simulink model "HDVPSG_DelayComp_NewRef_RealDrop_case1"  (R2019b)
settings: Solver=FixedStepDiscrete  StartTime=0.0  StopTime=28  FixedStep=UT.Ts_Veh  RelTol=1e-3
PostLoadFcn:
  | if any(exist('dsrtsu_mdlpostloadfcn', 'file') ~= 0), dsrtsu_mdlpostloadfcn('Execute', bdroot); end
InitFcn:
  | , if any(exist('dsmpb_private', 'file') ~= 0), dsmpb_private('dsmpb_mdlclblib', 'Init', bdroot); end,
values from neighbouring files (symbols this model uses):
  BETA_HDV_Leader = 50    [HDVPSG_DelayComp_NewRef_RealDrop_script_case1.m]
  BETA_PSG_Follower = 150    [HDVPSG_DelayComp_NewRef_RealDrop_script_case1.m]
  CtrlZone_Length = 250    [HDVPSG_DelayComp_NewRef_RealDrop_script_case1.m]
  DELTA_D_MIN = 5    [HDVPSG_DelayComp_NewRef_RealDrop_script_case1.m]
  DELTA_DR_MG_TCC = 15    [HDVPSG_DelayComp_NewRef_RealDrop_script_case1.m]
  HDV_AMAX = 1.3    [HDVPSG_DelayComp_NewRef_RealDrop_script_case1.m]
  HDV_AMIN = -2.5    [HDVPSG_DelayComp_NewRef_RealDrop_script_case1.m]
  HDV_first_v0 = 13    [HDVPSG_DelayComp_NewRef_RealDrop_script_case1.m]
  HDV_HighMu_D = 9    [HDVPSG_DelayComp_NewRef_RealDrop_script_case1.m]
  HDV_HighMu_I = 27    [HDVPSG_DelayComp_NewRef_RealDrop_script_case1.m]
  HDV_HighMu_P = 27    [HDVPSG_DelayComp_NewRef_RealDrop_script_case1.m]
  HDV_HighMu_TRFC = 0.7    [HDVPSG_DelayComp_NewRef_RealDrop_script_case1.m]
  HDV_last_v0 = 13    [HDVPSG_DelayComp_NewRef_RealDrop_script_case1.m]
  HDV_LowMu_D = 6    [HDVPSG_DelayComp_NewRef_RealDrop_script_case1.m]
  HDV_LowMu_I = 8    [HDVPSG_DelayComp_NewRef_RealDrop_script_case1.m]
  HDV_LowMu_P = 12    [HDVPSG_DelayComp_NewRef_RealDrop_script_case1.m]
  HDV_LowMu_TRFC = 0.6    [HDVPSG_DelayComp_NewRef_RealDrop_script_case1.m]
  Np_MPC = 20    [HDVPSG_DelayComp_NewRef_RealDrop_script_case1.m]
  PSG_AMAX = 3.2    [HDVPSG_DelayComp_NewRef_RealDrop_script_case1.m]
  PSG_AMIN = -6    [HDVPSG_DelayComp_NewRef_RealDrop_script_case1.m]
  PSG_end_v0 = 13    [HDVPSG_DelayComp_NewRef_RealDrop_script_case1.m]
  PSG_first_v0 = 13    [HDVPSG_DelayComp_NewRef_RealDrop_script_case1.m]
  PSG_HighMu_D = 15    [HDVPSG_DelayComp_NewRef_RealDrop_script_case1.m]
  PSG_HighMu_I = 125    [HDVPSG_DelayComp_NewRef_RealDrop_script_case1.m]
  PSG_HighMu_P = 75    [HDVPSG_DelayComp_NewRef_RealDrop_script_case1.m]
  PSG_HighMu_TRFC = 0.8    [HDVPSG_DelayComp_NewRef_RealDrop_script_case1.m]
  PSG_LowMu_D = 12    [HDVPSG_DelayComp_NewRef_RealDrop_script_case1.m]
  PSG_LowMu_I = 64    [HDVPSG_DelayComp_NewRef_RealDrop_script_case1.m]
  PSG_LowMu_P = 48    [HDVPSG_DelayComp_NewRef_RealDrop_script_case1.m]
  PSG_LowMu_TRFC = 0.7    [HDVPSG_DelayComp_NewRef_RealDrop_script_case1.m]
  PSG_middle_v0 = 13    [HDVPSG_DelayComp_NewRef_RealDrop_script_case1.m]
  Q_Leader = 1    [HDVPSG_DelayComp_NewRef_RealDrop_script_case1.m]
  Qd_dot_PSG_Follower = 2    [HDVPSG_DelayComp_NewRef_RealDrop_script_case1.m]
  Qd_PSG_Follower = 10    [HDVPSG_DelayComp_NewRef_RealDrop_script_case1.m]
  R_Leader = 20    [HDVPSG_DelayComp_NewRef_RealDrop_script_case1.m]
  R_PSG_Follower = 1    [HDVPSG_DelayComp_NewRef_RealDrop_script_case1.m]
  Recved_40_1 = Recved_Flag_Combined(47740,:)    [HDVPSG_DelayComp_NewRef_RealDrop_script_case1.m]
  Recved_40_2 = Recved_Flag_Combined(47780,:)    [HDVPSG_DelayComp_NewRef_RealDrop_script_case1.m]
  Recved_40_3 = Recved_Flag_Combined(49536,:)    [HDVPSG_DelayComp_NewRef_RealDrop_script_case1.m]
  Recved_40_4 = Recved_Flag_Combined(118106,:)    [HDVPSG_DelayComp_NewRef_RealDrop_script_case1.m]
  Rho_deltad_PSG_Follower = 1e3    (= 1000)    [HDVPSG_DelayComp_NewRef_RealDrop_script_case1.m]
  Rho_v_PSG_Follower = 1e3    (= 1000)    [HDVPSG_DelayComp_NewRef_RealDrop_script_case1.m]
  T_ADE = 0.01    [HDVPSG_DelayComp_NewRef_RealDrop_script_case1.m]
  V_MAX = 40    [HDVPSG_DelayComp_NewRef_RealDrop_script_case1.m]
  V_MIN = 0    [HDVPSG_DelayComp_NewRef_RealDrop_script_case1.m]
  VR_MG_TCC = 15    [HDVPSG_DelayComp_NewRef_RealDrop_script_case1.m]
undefined symbols (not defined in the file or in its folder): DiscIntNeverNeededParam, UT
libraries: simulink x46
(part 4 of 16)

== system HDVPSG_DelayComp_NewRef_RealDrop_case1/PSG2_control_withPDR_compen/Subsystem17 ==
  delta_dTCC : Inport
  T_end : Inport  Port=2
  veh0_dend_0 : Inport  Port=3
  veh2_dend_0 : Inport  Port=4
  veh0_v0 : Inport  Port=5
  veh2_v0 : Inport  Port=6
  Enable : EnablePort
  Add : Sum  Inputs=+-
  Add1 : Sum  Inputs=-+
  Poly_coefficient : MATLAB Function  TreatAsAtomicUnit=on
  a_0 : Outport
  a_1 : Outport  Port=2
  a_2 : Outport  Port=3
  a_3 : Outport  Port=4
  wires:
  Poly_coefficient/2(a_1) -> a_1/1
  Add/1 -> Poly_coefficient/1(delta_d0)
  Poly_coefficient/1(a_0) -> a_0/1
  T_end/1 -> Poly_coefficient/4(Tend)
  Add1/1 -> Poly_coefficient/3(delta_v0)  "delta_dr_dot"
  delta_dTCC/1 -> Poly_coefficient/2(delta_dTCC)
  Poly_coefficient/3(a_2) -> a_2/1
  Poly_coefficient/4(a_3) -> a_3/1
  veh0_dend_0/1 -> Add/2
  veh2_dend_0/1 -> Add/1
  veh2_v0/1 -> Add1/1
  veh0_v0/1 -> Add1/2

== system HDVPSG_DelayComp_NewRef_RealDrop_case1/PSG2_control_withPDR_compen/Subsystem18 ==
  a0 : Inport
  a1 : Inport  Port=2
  a2 : Inport  Port=3
  a3 : Inport  Port=4
  t_sumo : Inport  Port=5
  Ref : MATLAB Function  TreatAsAtomicUnit=on
  Ref_Pre_Vec : MATLAB Function  TreatAsAtomicUnit=on
  delta_dr : Outport
  delta_dr_dot : Outport  Port=2
  delta_dr_Pre_Vec : Outport  Port=3
  delta_dr_dot_Pre_Vec : Outport  Port=4
  wires:
  a2/1 -> Ref_Pre_Vec/3(a_2), Ref/3(a_2)
  Ref/2(delta_dr_dot) -> delta_dr_dot/1
  Ref/1(delta_dr) -> delta_dr/1
  t_sumo/1 -> Ref_Pre_Vec/5(t_sumo), Ref/5(t_sumo)
  a3/1 -> Ref_Pre_Vec/4(a_3), Ref/4(a_3)
  a1/1 -> Ref_Pre_Vec/2(a_1), Ref/2(a_1)
  a0/1 -> Ref_Pre_Vec/1(a_0), Ref/1(a_0)
  Ref_Pre_Vec/1(delta_dr_Pre_Vec) -> delta_dr_Pre_Vec/1
  Ref_Pre_Vec/2(delta_dr_dot_Pre_Vec) -> delta_dr_dot_Pre_Vec/1

== system HDVPSG_DelayComp_NewRef_RealDrop_case1/PSG2_control_withPDR_compen/Subsystem2 ==
  Lost_Step : Inport
  delta_d_pre_freeze_if_lost : Inport  Port=2
  delta_d_measure : Inport  Port=3
  Constant1 : Constant  Value=[1:1:Np_MPC+1]
  Lookup Table Dynamic : simulink/Lookup Tables/Lookup Table Dynamic  LookUpMeth=Interpolation-Extrapolation  OutDataType=fixdt('double')  OutScaling=[]  OutputDataTypeScalingMode=Specify via dialog  OutDataTypeStr=double  DoSatur=off
      settings: SourceProductName=Simulink
  MATLAB Function3 : MATLAB Function  TreatAsAtomicUnit=on
  Mux : Mux  Inputs=2
  Saturation : Saturate  UpperLimit=Np_MPC+1  LowerLimit=0
  Scope : Scope
  Switch : Switch  Criteria=u2 > Threshold  Threshold=Np_MPC+1
  delta_d_enhanced : Outport
  wires:
  delta_d_pre_freeze_if_lost/1 -> MATLAB Function3/2(delta_d_pre_freeze_if_lost), Lookup Table Dynamic/3
  delta_d_measure/1 -> MATLAB Function3/3(delta_d_measure)
  Constant1/1 -> Lookup Table Dynamic/2
  Lost_Step/1 -> Switch/2, Saturation/1, Lookup Table Dynamic/1
  Mux/1 -> Scope/1
  Switch/1 -> delta_d_enhanced/1
  Lookup Table Dynamic/1 -> Mux/1, Switch/1  "extrapolation_outside_Hp"
  MATLAB Function3/1(delta_d_MPC) -> Mux/2, Switch/3  "within Hp"
  Saturation/1 -> MATLAB Function3/1(Lost_Step)

== system HDVPSG_DelayComp_NewRef_RealDrop_case1/PSG2_control_withPDR_compen/Subsystem3 ==
  v_ego : Inport
  a_ego : Inport  Port=2
  t_all_leader : Inport  Port=3
  t_leader_has_run : Inport  Port=4
  Time_headway : Inport  Port=5
  t_PRE_has_run : Inport  Port=6
  Enable : EnablePort
  Add9 : Sum  Inputs=+-+
  v_ego_ini : Outport
  a_ego_ini : Outport  Port=2
  T_all_to_MP_ego : Outport  Port=3
  t_PRE_has_run_ini : Outport  Port=4
  wires:
  v_ego/1 -> v_ego_ini/1
  a_ego/1 -> a_ego_ini/1
  Add9/1 -> T_all_to_MP_ego/1
  t_leader_has_run/1 -> Add9/2
  Time_headway/1 -> Add9/3
  t_all_leader/1 -> Add9/1
  t_PRE_has_run/1 -> t_PRE_has_run_ini/1

== system HDVPSG_DelayComp_NewRef_RealDrop_case1/PSG3_control_withPDR_compen/Enabled and Triggered Subsystem ==
  delta_d_pre : Inport
  Enable : EnablePort
  delta_d_pre_freeze : Outport
  wires:
  delta_d_pre/1 -> delta_d_pre_freeze/1

== system HDVPSG_DelayComp_NewRef_RealDrop_case1/PSG3_control_withPDR_compen/Subsystem ==
  Recv : Inport
  Compare To Zero1 : simulink/Logic and Bit Operations/Compare To Zero  relop===  OutDataTypeStr=boolean
  Constant3 : Constant  Value=0
  Enabled and Triggered Subsystem1 : Subsystem  TreatAsAtomicUnit=on
  Switch : Switch  Criteria=u2 > Threshold
  Lost_Step : Outport
  wires:
  Switch/1 -> Lost_Step/1
  Recv/1 -> Compare To Zero1/1
  Constant3/1 -> Switch/3
  Enabled and Triggered Subsystem1/1(Lost_stop) -> Switch/1
  Compare To Zero1/1 -> Enabled and Triggered Subsystem1/Enable, Switch/2

== system HDVPSG_DelayComp_NewRef_RealDrop_case1/PSG3_control_withPDR_compen/Subsystem17 ==
  delta_dTCC : Inport
  T_end : Inport  Port=2
  veh0_dend_0 : Inport  Port=3
  veh2_dend_0 : Inport  Port=4
  veh0_v0 : Inport  Port=5
  veh2_v0 : Inport  Port=6
  Enable : EnablePort
  Add : Sum  Inputs=+-
  Add1 : Sum  Inputs=-+
  Poly_coefficient : MATLAB Function  TreatAsAtomicUnit=on
  a_0 : Outport
  a_1 : Outport  Port=2
  a_2 : Outport  Port=3
  a_3 : Outport  Port=4
  wires:
  veh0_v0/1 -> Add1/2
  veh2_v0/1 -> Add1/1
  veh2_dend_0/1 -> Add/1
  veh0_dend_0/1 -> Add/2
  Poly_coefficient/4(a_3) -> a_3/1
  Poly_coefficient/3(a_2) -> a_2/1
  delta_dTCC/1 -> Poly_coefficient/2(delta_dTCC)
  Add1/1 -> Poly_coefficient/3(delta_v0)  "delta_dr_dot"
  T_end/1 -> Poly_coefficient/4(Tend)
  Poly_coefficient/1(a_0) -> a_0/1
  Add/1 -> Poly_coefficient/1(delta_d0)
  Poly_coefficient/2(a_1) -> a_1/1

== system HDVPSG_DelayComp_NewRef_RealDrop_case1/PSG3_control_withPDR_compen/Subsystem18 ==
  a0 : Inport
  a1 : Inport  Port=2
  a2 : Inport  Port=3
  a3 : Inport  Port=4
  t_sumo : Inport  Port=5
  Ref : MATLAB Function  TreatAsAtomicUnit=on
  Ref_Pre_Vec : MATLAB Function  TreatAsAtomicUnit=on
  delta_dr : Outport
  delta_dr_dot : Outport  Port=2
  delta_dr_Pre_Vec : Outport  Port=3
  delta_dr_dot_Pre_Vec : Outport  Port=4
  wires:
  Ref_Pre_Vec/2(delta_dr_dot_Pre_Vec) -> delta_dr_dot_Pre_Vec/1
  Ref_Pre_Vec/1(delta_dr_Pre_Vec) -> delta_dr_Pre_Vec/1
  a0/1 -> Ref/1(a_0), Ref_Pre_Vec/1(a_0)
  a1/1 -> Ref/2(a_1), Ref_Pre_Vec/2(a_1)
  a3/1 -> Ref/4(a_3), Ref_Pre_Vec/4(a_3)
  t_sumo/1 -> Ref/5(t_sumo), Ref_Pre_Vec/5(t_sumo)
  Ref/1(delta_dr) -> delta_dr/1
  Ref/2(delta_dr_dot) -> delta_dr_dot/1
  a2/1 -> Ref/3(a_2), Ref_Pre_Vec/3(a_2)

== system HDVPSG_DelayComp_NewRef_RealDrop_case1/PSG3_control_withPDR_compen/Subsystem2 ==
  Lost_Step : Inport
  delta_d_pre_freeze_if_lost : Inport  Port=2
  delta_d_measure : Inport  Port=3
  Constant1 : Constant  Value=[1:1:Np_MPC+1]
  Lookup Table Dynamic : simulink/Lookup Tables/Lookup Table Dynamic  LookUpMeth=Interpolation-Extrapolation  OutDataType=fixdt('double')  OutScaling=[]  OutputDataTypeScalingMode=Specify via dialog  OutDataTypeStr=double  DoSatur=off
      settings: SourceProductName=Simulink
  MATLAB Function3 : MATLAB Function  TreatAsAtomicUnit=on
  Mux : Mux  Inputs=2
  Saturation : Saturate  UpperLimit=Np_MPC+1  LowerLimit=0
  Scope : Scope
  Switch : Switch  Criteria=u2 > Threshold  Threshold=Np_MPC+1
  delta_d_enhanced : Outport
  wires:
  delta_d_pre_freeze_if_lost/1 -> MATLAB Function3/2(delta_d_pre_freeze_if_lost), Lookup Table Dynamic/3
  delta_d_measure/1 -> MATLAB Function3/3(delta_d_measure)
  Constant1/1 -> Lookup Table Dynamic/2
  Lost_Step/1 -> Switch/2, Saturation/1, Lookup Table Dynamic/1
  Mux/1 -> Scope/1
  Switch/1 -> delta_d_enhanced/1
  Lookup Table Dynamic/1 -> Mux/1, Switch/1  "extrapolation_outside_Hp"
  MATLAB Function3/1(delta_d_MPC) -> Mux/2, Switch/3  "within Hp"
  Saturation/1 -> MATLAB Function3/1(Lost_Step)

== system HDVPSG_DelayComp_NewRef_RealDrop_case1/PSG3_control_withPDR_compen/Subsystem3 ==
  v_ego : Inport
  a_ego : Inport  Port=2
  t_all_leader : Inport  Port=3
  t_leader_has_run : Inport  Port=4
  Time_headway : Inport  Port=5
  t_PRE_has_run : Inport  Port=6
  Enable : EnablePort
  Add9 : Sum  Inputs=+-+
  v_ego_ini : Outport
  a_ego_ini : Outport  Port=2
  T_all_to_MP_ego : Outport  Port=3
  t_PRE_has_run_ini : Outport  Port=4
  wires:
  t_PRE_has_run/1 -> t_PRE_has_run_ini/1
  t_all_leader/1 -> Add9/1
  Time_headway/1 -> Add9/3
  t_leader_has_run/1 -> Add9/2
  Add9/1 -> T_all_to_MP_ego/1
  a_ego/1 -> a_ego_ini/1
  v_ego/1 -> v_ego_ini/1

== system HDVPSG_DelayComp_NewRef_RealDrop_case1/Subsystem1/PSG_first ==
  note: [v: 0--13--20]
      | High Frict PSG: P=75, I=125, D=15, TRFC=0.8 -->   -7.2<a<4.4
      | Low Frict  PSG: P=48, I=64,   D=12, TRFC=0.7 -->   -6.0<a<3.2
      |
      | High Frict HDV: P=27, I=27, D=9, TRFC=0.7 -->  -4.3<a<2.2
      | Low Frict  HDV: P=12, I=8,   D=6, TRFC=0.6 -->  -2.5<a<1.3
      |
      | ULMPC treat sudden drop of TRFC!
  vxr : Inport
  PID_P : Inport  Port=2
  PID_I : Inport  Port=3
  PID_D : Inport  Port=4
  TRFC : Inport  Port=5
  v_ini : Inport  Port=6
  Body Fixed Vehicle Dynamics : Subsystem
  Constant{1..5} (5 alike) : Constant  Value=0
  Cruise Speed Control : Subsystem
  Gain{,1..3} (4 alike) : Gain  Gain=UT.Rw
  Global Coordinates : Subsystem
  Scope : Scope
  Scope1 : Scope
  Scope3 : Scope
  Terminator : Terminator
  Vx : Scope
  X : Scope
  Y : Scope
  ax : Scope
  ay : Scope
  deg/rad : Gain  Gain=pi/180
  deg/rad1 : Gain  Gain=pi/180
  left/right wheel steer : Subsystem
  omegafl : Scope
  omegafr : Scope
  omegarl : Scope
  omegarr : Scope
  vy : Scope
  yaw : Scope
  yaw_rate : Scope
  vx : Outport
  wires:
  Constant4/1 -> Body Fixed Vehicle Dynamics/2(Brake)
  Constant3/1 -> Body Fixed Vehicle Dynamics/5(slope)
  Body Fixed Vehicle Dynamics/5(ax) -> ax/1
  Body Fixed Vehicle Dynamics/8(Yaw Angle) -> yaw/1, Global Coordinates/1(Heading Angle)
  left/right wheel steer/2(Left wheel steer ground (deg)) -> deg/rad/1
  left/right wheel steer/1(Right wheel steer ground (deg)) -> deg/rad1/1
  deg/rad1/1 -> Scope3/1, Body Fixed Vehicle Dynamics/3(deltaFR)
  Gain3/1 -> omegarr/1
  Global Coordinates/2(Y) -> Y/1
  Body Fixed Vehicle Dynamics/2(omegafr) -> Gain1/1
  Constant1/1 -> left/right wheel steer/1(steering wheel angle deg)
  deg/rad/1 -> Body Fixed Vehicle Dynamics/4(deltaFL)
  Body Fixed Vehicle Dynamics/11(Beta) -> Terminator/1
  Body Fixed Vehicle Dynamics/9(ay) -> ay/1
  Gain1/1 -> omegafr/1
  vxr/1 -> Cruise Speed Control/2(Vxr)
  Body Fixed Vehicle Dynamics/12(Sideslip Angle Alpha) -> Scope/1
  Body Fixed Vehicle Dynamics/7("Yaw Rate ") -> yaw_rate/1
  Gain/1 -> omegafl/1
  Gain2/1 -> omegarl/1
  Cruise Speed Control/1(Throttle) -> Body Fixed Vehicle Dynamics/1(Tdf), Scope1/1
  Body Fixed Vehicle Dynamics/10(Vy) -> Global Coordinates/3(Vy), vy/1
  Body Fixed Vehicle Dynamics/1(omegafl) -> Gain/1
  Body Fixed Vehicle Dynamics/4(omegarr) -> Gain3/1
  Body Fixed Vehicle Dynamics/3(omegarl) -> Gain2/1
  Body Fixed Vehicle Dynamics/6(Vx) -> Global Coordinates/2(Vx), Vx/1, Cruise Speed Control/1(Vx), vx/1
  Global Coordinates/1(X) -> X/1
  PID_P/1 -> Cruise Speed Control/3(PID_P)
  PID_I/1 -> Cruise Speed Control/4(PID_I)
  PID_D/1 -> Cruise Speed Control/5(PID_D)
  TRFC/1 -> Body Fixed Vehicle Dynamics/6(TRFC)
  v_ini/1 -> Body Fixed Vehicle Dynamics/7(V_ini)
  Constant2/1 -> Body Fixed Vehicle Dynamics/8(yaw_ini)
  Constant5/1 -> Body Fixed Vehicle Dynamics/9(vy_ini)

== system HDVPSG_DelayComp_NewRef_RealDrop_case1/Subsystem1/Subsystem4 ==
  Dist_to_MP : Inport
  Constant57 : Constant  Value=PSG_HighMu_P
  Constant58 : Constant  Value=PSG_LowMu_P
  MATLAB Function : MATLAB Function  TreatAsAtomicUnit=on
  Switch : Switch  Criteria=u2 > Threshold
  PSG_P : Outport
  HighMu : Outport  Port=2
  wires:
  MATLAB Function/1(HighTRFC) -> HighMu/1, Switch/2
  Dist_to_MP/1 -> MATLAB Function/1(distMP)
  Constant57/1 -> Switch/1
  Constant58/1 -> Switch/3
  Switch/1 -> PSG_P/1

== system HDVPSG_DelayComp_NewRef_RealDrop_case1/Subsystem1/Subsystem5 ==
  Dist_to_MP : Inport
  Constant57 : Constant  Value=PSG_HighMu_I
  Constant58 : Constant  Value=PSG_LowMu_I
  MATLAB Function : MATLAB Function  TreatAsAtomicUnit=on
  Switch : Switch  Criteria=u2 > Threshold
  PSG_I : Outport
  wires:
  Dist_to_MP/1 -> MATLAB Function/1(distMP)
  Switch/1 -> PSG_I/1
  Constant58/1 -> Switch/3
  Constant57/1 -> Switch/1
  MATLAB Function/1(HighTRFC) -> Switch/2

== system HDVPSG_DelayComp_NewRef_RealDrop_case1/Subsystem1/Subsystem6 ==
  Dist_to_MP : Inport
  Constant57 : Constant  Value=PSG_HighMu_D
  Constant58 : Constant  Value=PSG_LowMu_D
  MATLAB Function : MATLAB Function  TreatAsAtomicUnit=on
  Switch : Switch  Criteria=u2 > Threshold
  PSG_D : Outport
  wires:
  Dist_to_MP/1 -> MATLAB Function/1(distMP)
  Constant57/1 -> Switch/1
  Constant58/1 -> Switch/3
  Switch/1 -> PSG_D/1
  MATLAB Function/1(HighTRFC) -> Switch/2

== system HDVPSG_DelayComp_NewRef_RealDrop_case1/Subsystem1/Subsystem7 ==
  Dist_to_MP : Inport
  Constant1 : Constant  Value=PSG_LowMu_TRFC
  Constant57 : Constant  Value=PSG_HighMu_TRFC
  MATLAB Function : MATLAB Function  TreatAsAtomicUnit=on
  Switch : Switch  Criteria=u2 > Threshold
  PSG_Mu : Outport
  wires:
  Dist_to_MP/1 -> MATLAB Function/1(distMP)
  Switch/1 -> PSG_Mu/1
  Constant1/1 -> Switch/3
  Constant57/1 -> Switch/1
  MATLAB Function/1(HighTRFC) -> Switch/2

== system HDVPSG_DelayComp_NewRef_RealDrop_case1/Subsystem12/ARE_First_Order_Derivative_[1,0,0]5 ==
  a : Inport
  Trigger : TriggerPort  TriggerType=either  VariantControl=Variant  ZeroCross=off  PortDimensions=1
  Constant : Constant  Value=T_ADE
  Constant52 : Constant  Value=0
  MATLAB Function : MATLAB Function  TreatAsAtomicUnit=on
  a_dot_hat : Outport  VectorParamsAs1DForOutWhenUnconnected=off
  wires:
  Constant52/1 -> MATLAB Function/3(u_init)
  a/1 -> MATLAB Function/1(U)
  MATLAB Function/1(Dot_U) -> a_dot_hat/1
  Constant/1 -> MATLAB Function/2(Ts)

== system HDVPSG_DelayComp_NewRef_RealDrop_case1/Subsystem15/Enabled Subsystem1 ==
  Front_to_end : Inport
  Enable : EnablePort
  Front_to_end_PDR : Outport
  wires:
  Front_to_end/1 -> Front_to_end_PDR/1

== system HDVPSG_DelayComp_NewRef_RealDrop_case1/Subsystem15/Enabled Subsystem2 ==
  v_Front : Inport
  Enable : EnablePort
  v_Front_PDR : Outport
  wires:
  v_Front/1 -> v_Front_PDR/1

== system HDVPSG_DelayComp_NewRef_RealDrop_case1/Subsystem15/Enabled Subsystem3 ==
  a_Front : Inport
  Enable : EnablePort
  a_Front_PDR : Outport
  wires:
  a_Front/1 -> a_Front_PDR/1

== system HDVPSG_DelayComp_NewRef_RealDrop_case1/Subsystem2/PSG_first ==
  note: [v: 0--13--20]
      | High Frict PSG: P=75, I=125, D=15, TRFC=0.8 -->   -7.2<a<4.4
      | Low Frict  PSG: P=48, I=64,   D=12, TRFC=0.7 -->   -6.0<a<3.2
      |
      | High Frict HDV: P=27, I=27, D=9, TRFC=0.7 -->  -4.3<a<2.2
      | Low Frict  HDV: P=12, I=8,   D=6, TRFC=0.6 -->  -2.5<a<1.3
      |
      | ULMPC treat sudden drop of TRFC!
  vxr : Inport
  PID_P : Inport  Port=2
  PID_I : Inport  Port=3
  PID_D : Inport  Port=4
  TRFC : Inport  Port=5
  v_ini : Inport  Port=6
  Body Fixed Vehicle Dynamics : Subsystem
  Constant{1..5} (5 alike) : Constant  Value=0
  Cruise Speed Control : Subsystem
  Gain{,1..3} (4 alike) : Gain  Gain=UT.Rw
  Global Coordinates : Subsystem
  Scope : Scope
  Scope1 : Scope
  Scope3 : Scope
  Terminator : Terminator
  Vx : Scope
  X : Scope
  Y : Scope
  ax : Scope
  ay : Scope
  deg/rad : Gain  Gain=pi/180
  deg/rad1 : Gain  Gain=pi/180
  left/right wheel steer : Subsystem
  omegafl : Scope
  omegafr : Scope
  omegarl : Scope
  omegarr : Scope
  vy : Scope
  yaw : Scope
  yaw_rate : Scope
  vx : Outport
  wires:
  Constant5/1 -> Body Fixed Vehicle Dynamics/9(vy_ini)
  Constant2/1 -> Body Fixed Vehicle Dynamics/8(yaw_ini)
  v_ini/1 -> Body Fixed Vehicle Dynamics/7(V_ini)
  TRFC/1 -> Body Fixed Vehicle Dynamics/6(TRFC)
  PID_D/1 -> Cruise Speed Control/5(PID_D)
  PID_I/1 -> Cruise Speed Control/4(PID_I)
  PID_P/1 -> Cruise Speed Control/3(PID_P)
  Global Coordinates/1(X) -> X/1
  Body Fixed Vehicle Dynamics/6(Vx) -> vx/1, Cruise Speed Control/1(Vx), Vx/1, Global Coordinates/2(Vx)
  Body Fixed Vehicle Dynamics/3(omegarl) -> Gain2/1
  Body Fixed Vehicle Dynamics/4(omegarr) -> Gain3/1
  Body Fixed Vehicle Dynamics/1(omegafl) -> Gain/1
  Body Fixed Vehicle Dynamics/10(Vy) -> vy/1, Global Coordinates/3(Vy)
  Cruise Speed Control/1(Throttle) -> Scope1/1, Body Fixed Vehicle Dynamics/1(Tdf)
  Gain2/1 -> omegarl/1
  Gain/1 -> omegafl/1
  Body Fixed Vehicle Dynamics/7("Yaw Rate ") -> yaw_rate/1
  Body Fixed Vehicle Dynamics/12(Sideslip Angle Alpha) -> Scope/1
  vxr/1 -> Cruise Speed Control/2(Vxr)
  Gain1/1 -> omegafr/1
  Body Fixed Vehicle Dynamics/9(ay) -> ay/1
  Body Fixed Vehicle Dynamics/11(Beta) -> Terminator/1
  deg/rad/1 -> Body Fixed Vehicle Dynamics/4(deltaFL)
  Constant1/1 -> left/right wheel steer/1(steering wheel angle deg)
  Body Fixed Vehicle Dynamics/2(omegafr) -> Gain1/1
  Global Coordinates/2(Y) -> Y/1
  Gain3/1 -> omegarr/1
  deg/rad1/1 -> Body Fixed Vehicle Dynamics/3(deltaFR), Scope3/1
  left/right wheel steer/1(Right wheel steer ground (deg)) -> deg/rad1/1
  left/right wheel steer/2(Left wheel steer ground (deg)) -> deg/rad/1
  Body Fixed Vehicle Dynamics/8(Yaw Angle) -> Global Coordinates/1(Heading Angle), yaw/1
  Body Fixed Vehicle Dynamics/5(ax) -> ax/1
  Constant3/1 -> Body Fixed Vehicle Dynamics/5(slope)
  Constant4/1 -> Body Fixed Vehicle Dynamics/2(Brake)

== system HDVPSG_DelayComp_NewRef_RealDrop_case1/Subsystem2/Subsystem4 ==
  Dist_to_MP : Inport
  Constant57 : Constant  Value=PSG_HighMu_P
  Constant58 : Constant  Value=PSG_LowMu_P
  MATLAB Function : MATLAB Function  TreatAsAtomicUnit=on
  Switch : Switch  Criteria=u2 > Threshold
  PSG_P : Outport
  HighMu : Outport  Port=2
  wires:
  Switch/1 -> PSG_P/1
  Constant58/1 -> Switch/3
  Constant57/1 -> Switch/1
  Dist_to_MP/1 -> MATLAB Function/1(distMP)
  MATLAB Function/1(HighTRFC) -> HighMu/1, Switch/2

== system HDVPSG_DelayComp_NewRef_RealDrop_case1/Subsystem2/Subsystem5 ==
  Dist_to_MP : Inport
  Constant57 : Constant  Value=PSG_HighMu_I
  Constant58 : Constant  Value=PSG_LowMu_I
  MATLAB Function : MATLAB Function  TreatAsAtomicUnit=on
  Switch : Switch  Criteria=u2 > Threshold
  PSG_I : Outport
  wires:
  Constant57/1 -> Switch/1
  Constant58/1 -> Switch/3
  Switch/1 -> PSG_I/1
  Dist_to_MP/1 -> MATLAB Function/1(distMP)
  MATLAB Function/1(HighTRFC) -> Switch/2

== system HDVPSG_DelayComp_NewRef_RealDrop_case1/Subsystem2/Subsystem6 ==
  Dist_to_MP : Inport
  Constant57 : Constant  Value=PSG_HighMu_D
  Constant58 : Constant  Value=PSG_LowMu_D
  MATLAB Function : MATLAB Function  TreatAsAtomicUnit=on
  Switch : Switch  Criteria=u2 > Threshold
  PSG_D : Outport
  wires:
  Switch/1 -> PSG_D/1
  Constant58/1 -> Switch/3
  Constant57/1 -> Switch/1
  Dist_to_MP/1 -> MATLAB Function/1(distMP)
  MATLAB Function/1(HighTRFC) -> Switch/2

== system HDVPSG_DelayComp_NewRef_RealDrop_case1/Subsystem2/Subsystem7 ==
  Dist_to_MP : Inport
  Constant1 : Constant  Value=PSG_LowMu_TRFC
  Constant57 : Constant  Value=PSG_HighMu_TRFC
  MATLAB Function : MATLAB Function  TreatAsAtomicUnit=on
  Switch : Switch  Criteria=u2 > Threshold
  PSG_Mu : Outport
  wires:
  Constant57/1 -> Switch/1
  Constant1/1 -> Switch/3
  Switch/1 -> PSG_Mu/1
  Dist_to_MP/1 -> MATLAB Function/1(distMP)
  MATLAB Function/1(HighTRFC) -> Switch/2

== system HDVPSG_DelayComp_NewRef_RealDrop_case1/Subsystem29/PSG_first ==
  note: [v: 0--13--20]
      | High Frict PSG: P=75, I=125, D=15, TRFC=0.8 -->   -7.2<a<4.4
      | Low Frict  PSG: P=48, I=64,   D=12, TRFC=0.7 -->   -6.0<a<3.2
      |
      | High Frict HDV: P=27, I=27, D=9, TRFC=0.7 -->  -4.3<a<2.2
      | Low Frict  HDV: P=12, I=8,   D=6, TRFC=0.6 -->  -2.5<a<1.3
      |
      | ULMPC treat sudden drop of TRFC!
  vxr : Inport
  PID_P : Inport  Port=2
  PID_I : Inport  Port=3
  PID_D : Inport  Port=4
  TRFC : Inport  Port=5
  v_ini : Inport  Port=6
  Body Fixed Vehicle Dynamics : Subsystem
  Constant{1..5} (5 alike) : Constant  Value=0
  Cruise Speed Control : Subsystem
  Gain{,1..3} (4 alike) : Gain  Gain=UT.Rw
  Global Coordinates : Subsystem
  Scope : Scope
  Scope1 : Scope
  Scope3 : Scope
  Terminator : Terminator
  Vx : Scope
  X : Scope
  Y : Scope
  ax : Scope
  ay : Scope
  deg/rad : Gain  Gain=pi/180
  deg/rad1 : Gain  Gain=pi/180
  left/right wheel steer : Subsystem
  omegafl : Scope
  omegafr : Scope
  omegarl : Scope
  omegarr : Scope
  vy : Scope
  yaw : Scope
  yaw_rate : Scope
  vx : Outport
  wires:
  Constant5/1 -> Body Fixed Vehicle Dynamics/9(vy_ini)
  Constant2/1 -> Body Fixed Vehicle Dynamics/8(yaw_ini)
  v_ini/1 -> Body Fixed Vehicle Dynamics/7(V_ini)
  TRFC/1 -> Body Fixed Vehicle Dynamics/6(TRFC)
  PID_D/1 -> Cruise Speed Control/5(PID_D)
  PID_I/1 -> Cruise Speed Control/4(PID_I)
  PID_P/1 -> Cruise Speed Control/3(PID_P)
  Global Coordinates/1(X) -> X/1
  Body Fixed Vehicle Dynamics/6(Vx) -> vx/1, Cruise Speed Control/1(Vx), Vx/1, Global Coordinates/2(Vx)
  Body Fixed Vehicle Dynamics/3(omegarl) -> Gain2/1
  Body Fixed Vehicle Dynamics/4(omegarr) -> Gain3/1
  Body Fixed Vehicle Dynamics/1(omegafl) -> Gain/1
  Body Fixed Vehicle Dynamics/10(Vy) -> vy/1, Global Coordinates/3(Vy)
  Cruise Speed Control/1(Throttle) -> Scope1/1, Body Fixed Vehicle Dynamics/1(Tdf)
  Gain2/1 -> omegarl/1
  Gain/1 -> omegafl/1
  Body Fixed Vehicle Dynamics/7("Yaw Rate ") -> yaw_rate/1
  Body Fixed Vehicle Dynamics/12(Sideslip Angle Alpha) -> Scope/1
  vxr/1 -> Cruise Speed Control/2(Vxr)
  Gain1/1 -> omegafr/1
  Body Fixed Vehicle Dynamics/9(ay) -> ay/1
  Body Fixed Vehicle Dynamics/11(Beta) -> Terminator/1
  deg/rad/1 -> Body Fixed Vehicle Dynamics/4(deltaFL)
  Constant1/1 -> left/right wheel steer/1(steering wheel angle deg)
  Body Fixed Vehicle Dynamics/2(omegafr) -> Gain1/1
  Global Coordinates/2(Y) -> Y/1
  Gain3/1 -> omegarr/1
  deg/rad1/1 -> Body Fixed Vehicle Dynamics/3(deltaFR), Scope3/1
  left/right wheel steer/1(Right wheel steer ground (deg)) -> deg/rad1/1
  left/right wheel steer/2(Left wheel steer ground (deg)) -> deg/rad/1
  Body Fixed Vehicle Dynamics/8(Yaw Angle) -> Global Coordinates/1(Heading Angle), yaw/1
  Body Fixed Vehicle Dynamics/5(ax) -> ax/1
  Constant3/1 -> Body Fixed Vehicle Dynamics/5(slope)
  Constant4/1 -> Body Fixed Vehicle Dynamics/2(Brake)

== system HDVPSG_DelayComp_NewRef_RealDrop_case1/Subsystem29/Subsystem4 ==
  Dist_to_MP : Inport
  Constant57 : Constant  Value=PSG_HighMu_P
  Constant58 : Constant  Value=PSG_LowMu_P
  MATLAB Function : MATLAB Function  TreatAsAtomicUnit=on
  Switch : Switch  Criteria=u2 > Threshold
  PSG_P : Outport
  HighMu : Outport  Port=2
  wires:
  Switch/1 -> PSG_P/1
  Constant58/1 -> Switch/3
  Constant57/1 -> Switch/1
  Dist_to_MP/1 -> MATLAB Function/1(distMP)
  MATLAB Function/1(HighTRFC) -> HighMu/1, Switch/2

== system HDVPSG_DelayComp_NewRef_RealDrop_case1/Subsystem29/Subsystem5 ==
  Dist_to_MP : Inport
  Constant57 : Constant  Value=PSG_HighMu_I
  Constant58 : Constant  Value=PSG_LowMu_I
  MATLAB Function : MATLAB Function  TreatAsAtomicUnit=on
  Switch : Switch  Criteria=u2 > Threshold
  PSG_I : Outport
  wires:
  Constant57/1 -> Switch/1
  Constant58/1 -> Switch/3
  Switch/1 -> PSG_I/1
  Dist_to_MP/1 -> MATLAB Function/1(distMP)
  MATLAB Function/1(HighTRFC) -> Switch/2

== system HDVPSG_DelayComp_NewRef_RealDrop_case1/Subsystem29/Subsystem6 ==
  Dist_to_MP : Inport
  Constant57 : Constant  Value=PSG_HighMu_D
  Constant58 : Constant  Value=PSG_LowMu_D
  MATLAB Function : MATLAB Function  TreatAsAtomicUnit=on
  Switch : Switch  Criteria=u2 > Threshold
  PSG_D : Outport
  wires:
  Switch/1 -> PSG_D/1
  Constant58/1 -> Switch/3
  Constant57/1 -> Switch/1
  Dist_to_MP/1 -> MATLAB Function/1(distMP)
  MATLAB Function/1(HighTRFC) -> Switch/2

== system HDVPSG_DelayComp_NewRef_RealDrop_case1/Subsystem29/Subsystem7 ==
  Dist_to_MP : Inport
  Constant1 : Constant  Value=PSG_LowMu_TRFC
  Constant57 : Constant  Value=PSG_HighMu_TRFC
  MATLAB Function : MATLAB Function  TreatAsAtomicUnit=on
  Switch : Switch  Criteria=u2 > Threshold
  PSG_Mu : Outport
  wires:
  Constant57/1 -> Switch/1
  Constant1/1 -> Switch/3
  Switch/1 -> PSG_Mu/1
  Dist_to_MP/1 -> MATLAB Function/1(distMP)
  MATLAB Function/1(HighTRFC) -> Switch/2

== system HDVPSG_DelayComp_NewRef_RealDrop_case1/Subsystem3/HDV_first ==
  note: [v: 0--13--20]
      | High Frict PSG: P=75, I=125, D=15, TRFC=0.8 -->   -7.2<a<4.4
      | Low Frict  PSG: P=48, I=64,   D=12, TRFC=0.7 -->   -6.0<a<3.2
      |
      | High Frict HDV: P=27, I=27, D=9, TRFC=0.7 -->  -4.3<a<2.2
      | Low Frict  HDV: P=12, I=8,   D=6, TRFC=0.6 -->  -2.5<a<1.3
      |
      | ULMPC treat sudden drop of TRFC!
  vxr : Inport
  PID_P : Inport  Port=2
  PID_I : Inport  Port=3
  PID_D : Inport  Port=4
  TRFC : Inport  Port=5
  v_ini : Inport  Port=6
  Body Fixed Vehicle Dynamics : Subsystem
  Constant{1..5} (5 alike) : Constant  Value=0
  Cruise Speed Control : Subsystem
  Gain{,1..3} (4 alike) : Gain  Gain=UT.Rw
  Global Coordinates : Subsystem
  Scope : Scope
  Scope1 : Scope
  Scope3 : Scope
  Terminator : Terminator
  Vx : Scope
  X : Scope
  Y : Scope
  ax : Scope
  ay : Scope
  deg/rad : Gain  Gain=pi/180
  deg/rad1 : Gain  Gain=pi/180
  left/right wheel steer : Subsystem
  omegafl : Scope
  omegafr : Scope
  omegarl : Scope
  omegarr : Scope
  vy : Scope
  yaw : Scope
  yaw_rate : Scope
  vx : Outport
  wires:
  Constant5/1 -> Body Fixed Vehicle Dynamics/9(vy_ini)
  Constant2/1 -> Body Fixed Vehicle Dynamics/8(yaw_ini)
  v_ini/1 -> Body Fixed Vehicle Dynamics/7(V_ini)
  TRFC/1 -> Body Fixed Vehicle Dynamics/6(TRFC)
  PID_D/1 -> Cruise Speed Control/5(PID_D)
  PID_I/1 -> Cruise Speed Control/4(PID_I)
  PID_P/1 -> Cruise Speed Control/3(PID_P)
  Global Coordinates/1(X) -> X/1
  Body Fixed Vehicle Dynamics/6(Vx) -> vx/1, Cruise Speed Control/1(Vx), Vx/1, Global Coordinates/2(Vx)
  Body Fixed Vehicle Dynamics/3(omegarl) -> Gain2/1
  Body Fixed Vehicle Dynamics/4(omegarr) -> Gain3/1
  Body Fixed Vehicle Dynamics/1(omegafl) -> Gain/1
  Body Fixed Vehicle Dynamics/10(Vy) -> vy/1, Global Coordinates/3(Vy)
  Cruise Speed Control/1(Throttle) -> Scope1/1, Body Fixed Vehicle Dynamics/1(Tdf)
  Gain2/1 -> omegarl/1
  Gain/1 -> omegafl/1
  Body Fixed Vehicle Dynamics/7("Yaw Rate ") -> yaw_rate/1
  Body Fixed Vehicle Dynamics/12(Sideslip Angle Alpha) -> Scope/1
  vxr/1 -> Cruise Speed Control/2(Vxr)
  Gain1/1 -> omegafr/1
  Body Fixed Vehicle Dynamics/9(ay) -> ay/1
  Body Fixed Vehicle Dynamics/11(Beta) -> Terminator/1
  deg/rad/1 -> Body Fixed Vehicle Dynamics/4(deltaFL)
  Constant1/1 -> left/right wheel steer/1(steering wheel angle deg)
  Body Fixed Vehicle Dynamics/2(omegafr) -> Gain1/1
  Global Coordinates/2(Y) -> Y/1
  Gain3/1 -> omegarr/1
  deg/rad1/1 -> Body Fixed Vehicle Dynamics/3(deltaFR), Scope3/1
  left/right wheel steer/1(Right wheel steer ground (deg)) -> deg/rad1/1
  left/right wheel steer/2(Left wheel steer ground (deg)) -> deg/rad/1
  Body Fixed Vehicle Dynamics/8(Yaw Angle) -> Global Coordinates/1(Heading Angle), yaw/1
  Body Fixed Vehicle Dynamics/5(ax) -> ax/1
  Constant3/1 -> Body Fixed Vehicle Dynamics/5(slope)
  Constant4/1 -> Body Fixed Vehicle Dynamics/2(Brake)

== system HDVPSG_DelayComp_NewRef_RealDrop_case1/Subsystem3/Subsystem16 ==
  Dist_to_MP : Inport
  Constant57 : Constant  Value=HDV_HighMu_P
  Constant58 : Constant  Value=HDV_LowMu_P
  MATLAB Function : MATLAB Function  TreatAsAtomicUnit=on
  Switch : Switch  Criteria=u2 > Threshold
  HDV_P : Outport
  HighMu : Outport  Port=2
  wires:
  Dist_to_MP/1 -> MATLAB Function/1(distMP)
  Constant58/1 -> Switch/3
  MATLAB Function/1(HighTRFC) -> HighMu/1, Switch/2
  Constant57/1 -> Switch/1
  Switch/1 -> HDV_P/1

== system HDVPSG_DelayComp_NewRef_RealDrop_case1/Subsystem3/Subsystem17 ==
  Dist_to_MP : Inport
  Constant57 : Constant  Value=HDV_HighMu_I
  Constant58 : Constant  Value=HDV_LowMu_I
  MATLAB Function : MATLAB Function  TreatAsAtomicUnit=on
  Switch : Switch  Criteria=u2 > Threshold
  HDV_I : Outport
  wires:
  MATLAB Function/1(HighTRFC) -> Switch/2
  Dist_to_MP/1 -> MATLAB Function/1(distMP)
  Constant58/1 -> Switch/3
  Constant57/1 -> Switch/1
  Switch/1 -> HDV_I/1

== system HDVPSG_DelayComp_NewRef_RealDrop_case1/Subsystem3/Subsystem18 ==
  Dist_to_MP : Inport
  Constant57 : Constant  Value=HDV_HighMu_D
  Constant58 : Constant  Value=HDV_LowMu_D
  MATLAB Function : MATLAB Function  TreatAsAtomicUnit=on
  Switch : Switch  Criteria=u2 > Threshold
  HDV_D : Outport
  wires:
  MATLAB Function/1(HighTRFC) -> Switch/2
  Dist_to_MP/1 -> MATLAB Function/1(distMP)
  Constant58/1 -> Switch/3
  Constant57/1 -> Switch/1
  Switch/1 -> HDV_D/1

== system HDVPSG_DelayComp_NewRef_RealDrop_case1/Subsystem3/Subsystem7 ==
  Dist_to_MP : Inport
  Constant1 : Constant  Value=HDV_LowMu_TRFC
  Constant57 : Constant  Value=HDV_HighMu_TRFC
  MATLAB Function : MATLAB Function  TreatAsAtomicUnit=on
  Switch : Switch  Criteria=u2 > Threshold
  HDV_Mu : Outport
  wires:
  MATLAB Function/1(HighTRFC) -> Switch/2
  Dist_to_MP/1 -> MATLAB Function/1(distMP)
  Constant1/1 -> Switch/3
  Constant57/1 -> Switch/1
  Switch/1 -> HDV_Mu/1

== system HDVPSG_DelayComp_NewRef_RealDrop_case1/Subsystem4/Enabled Subsystem1 ==
  Front_to_end : Inport
  Enable : EnablePort
  Front_to_end_PDR : Outport
  wires:
  Front_to_end/1 -> Front_to_end_PDR/1

== system HDVPSG_DelayComp_NewRef_RealDrop_case1/Subsystem4/Enabled Subsystem2 ==
  v_Front : Inport
  Enable : EnablePort
  v_Front_PDR : Outport
  wires:
  v_Front/1 -> v_Front_PDR/1

== system HDVPSG_DelayComp_NewRef_RealDrop_case1/Subsystem4/Enabled Subsystem3 ==
  a_Front : Inport
  Enable : EnablePort
  a_Front_PDR : Outport
  wires:
  a_Front/1 -> a_Front_PDR/1

== system HDVPSG_DelayComp_NewRef_RealDrop_case1/Subsystem5/Enabled Subsystem1 ==
  Front_to_end : Inport
  Enable : EnablePort
  Front_to_end_PDR : Outport
  wires:
  Front_to_end/1 -> Front_to_end_PDR/1

== system HDVPSG_DelayComp_NewRef_RealDrop_case1/Subsystem5/Enabled Subsystem2 ==
  v_Front : Inport
  Enable : EnablePort
  v_Front_PDR : Outport
  wires:
  v_Front/1 -> v_Front_PDR/1

== system HDVPSG_DelayComp_NewRef_RealDrop_case1/Subsystem5/Enabled Subsystem3 ==
  a_Front : Inport
  Enable : EnablePort
  a_Front_PDR : Outport
  wires:
  a_Front/1 -> a_Front_PDR/1

== system HDVPSG_DelayComp_NewRef_RealDrop_case1/Subsystem6/HDV_first ==
  note: [v: 0--13--20]
      | High Frict PSG: P=75, I=125, D=15, TRFC=0.8 -->   -7.2<a<4.4
      | Low Frict  PSG: P=48, I=64,   D=12, TRFC=0.7 -->   -6.0<a<3.2
      |
      | High Frict HDV: P=27, I=27, D=9, TRFC=0.7 -->  -4.3<a<2.2
      | Low Frict  HDV: P=12, I=8,   D=6, TRFC=0.6 -->  -2.5<a<1.3
      |
      | ULMPC treat sudden drop of TRFC!
  vxr : Inport
  PID_P : Inport  Port=2
  PID_I : Inport  Port=3
  PID_D : Inport  Port=4
  TRFC : Inport  Port=5
  v_ini : Inport  Port=6
  Body Fixed Vehicle Dynamics : Subsystem
  Constant{1..5} (5 alike) : Constant  Value=0
  Cruise Speed Control : Subsystem
  Gain{,1..3} (4 alike) : Gain  Gain=UT.Rw
  Global Coordinates : Subsystem
  Scope : Scope
  Scope1 : Scope
  Scope3 : Scope
  Terminator : Terminator
  Vx : Scope
  X : Scope
  Y : Scope
  ax : Scope
  ay : Scope
  deg/rad : Gain  Gain=pi/180
  deg/rad1 : Gain  Gain=pi/180
  left/right wheel steer : Subsystem
  omegafl : Scope
  omegafr : Scope
  omegarl : Scope
  omegarr : Scope
  vy : Scope
  yaw : Scope
  yaw_rate : Scope
  vx : Outport
  wires:
  Constant4/1 -> Body Fixed Vehicle Dynamics/2(Brake)
  Constant3/1 -> Body Fixed Vehicle Dynamics/5(slope)
  Body Fixed Vehicle Dynamics/5(ax) -> ax/1
  Body Fixed Vehicle Dynamics/8(Yaw Angle) -> yaw/1, Global Coordinates/1(Heading Angle)
  left/right wheel steer/2(Left wheel steer ground (deg)) -> deg/rad/1
  left/right wheel steer/1(Right wheel steer ground (deg)) -> deg/rad1/1
  deg/rad1/1 -> Scope3/1, Body Fixed Vehicle Dynamics/3(deltaFR)
  Gain3/1 -> omegarr/1
  Global Coordinates/2(Y) -> Y/1
  Body Fixed Vehicle Dynamics/2(omegafr) -> Gain1/1
  Constant1/1 -> left/right wheel steer/1(steering wheel angle deg)
  deg/rad/1 -> Body Fixed Vehicle Dynamics/4(deltaFL)
  Body Fixed Vehicle Dynamics/11(Beta) -> Terminator/1
  Body Fixed Vehicle Dynamics/9(ay) -> ay/1
  Gain1/1 -> omegafr/1
  vxr/1 -> Cruise Speed Control/2(Vxr)
  Body Fixed Vehicle Dynamics/12(Sideslip Angle Alpha) -> Scope/1
  Body Fixed Vehicle Dynamics/7("Yaw Rate ") -> yaw_rate/1
  Gain/1 -> omegafl/1
  Gain2/1 -> omegarl/1
  Cruise Speed Control/1(Throttle) -> Body Fixed Vehicle Dynamics/1(Tdf), Scope1/1
  Body Fixed Vehicle Dynamics/10(Vy) -> Global Coordinates/3(Vy), vy/1
  Body Fixed Vehicle Dynamics/1(omegafl) -> Gain/1
  Body Fixed Vehicle Dynamics/4(omegarr) -> Gain3/1
  Body Fixed Vehicle Dynamics/3(omegarl) -> Gain2/1
  Body Fixed Vehicle Dynamics/6(Vx) -> Global Coordinates/2(Vx), Vx/1, Cruise Speed Control/1(Vx), vx/1
  Global Coordinates/1(X) -> X/1
  PID_P/1 -> Cruise Speed Control/3(PID_P)
  PID_I/1 -> Cruise Speed Control/4(PID_I)
  PID_D/1 -> Cruise Speed Control/5(PID_D)
  TRFC/1 -> Body Fixed Vehicle Dynamics/6(TRFC)
  v_ini/1 -> Body Fixed Vehicle Dynamics/7(V_ini)
  Constant2/1 -> Body Fixed Vehicle Dynamics/8(yaw_ini)
  Constant5/1 -> Body Fixed Vehicle Dynamics/9(vy_ini)

== system HDVPSG_DelayComp_NewRef_RealDrop_case1/Subsystem6/Subsystem16 ==
  Dist_to_MP : Inport
  Constant57 : Constant  Value=HDV_HighMu_P
  Constant58 : Constant  Value=HDV_LowMu_P
  MATLAB Function : MATLAB Function  TreatAsAtomicUnit=on
  Switch : Switch  Criteria=u2 > Threshold
  HDV_P : Outport
  HighMu : Outport  Port=2
  wires:
  Constant58/1 -> Switch/3
  Dist_to_MP/1 -> MATLAB Function/1(distMP)
  MATLAB Function/1(HighTRFC) -> Switch/2, HighMu/1
  Constant57/1 -> Switch/1
  Switch/1 -> HDV_P/1

== system HDVPSG_DelayComp_NewRef_RealDrop_case1/Subsystem6/Subsystem17 ==
  Dist_to_MP : Inport
  Constant57 : Constant  Value=HDV_HighMu_I
  Constant58 : Constant  Value=HDV_LowMu_I
  MATLAB Function : MATLAB Function  TreatAsAtomicUnit=on
  Switch : Switch  Criteria=u2 > Threshold
  HDV_I : Outport
  wires:
  Constant58/1 -> Switch/3
  Dist_to_MP/1 -> MATLAB Function/1(distMP)
  MATLAB Function/1(HighTRFC) -> Switch/2
  Constant57/1 -> Switch/1
  Switch/1 -> HDV_I/1

== system HDVPSG_DelayComp_NewRef_RealDrop_case1/Subsystem6/Subsystem18 ==
  Dist_to_MP : Inport
  Constant57 : Constant  Value=HDV_HighMu_D
  Constant58 : Constant  Value=HDV_LowMu_D
  MATLAB Function : MATLAB Function  TreatAsAtomicUnit=on
  Switch : Switch  Criteria=u2 > Threshold
  HDV_D : Outport
  wires:
  Constant58/1 -> Switch/3
  Dist_to_MP/1 -> MATLAB Function/1(distMP)
  MATLAB Function/1(HighTRFC) -> Switch/2
  Constant57/1 -> Switch/1
  Switch/1 -> HDV_D/1

== system HDVPSG_DelayComp_NewRef_RealDrop_case1/Subsystem6/Subsystem7 ==
  Dist_to_MP : Inport
  Constant1 : Constant  Value=HDV_LowMu_TRFC
  Constant57 : Constant  Value=HDV_HighMu_TRFC
  MATLAB Function : MATLAB Function  TreatAsAtomicUnit=on
  Switch : Switch  Criteria=u2 > Threshold
  HDV_Mu : Outport
  wires:
  Constant1/1 -> Switch/3
  Dist_to_MP/1 -> MATLAB Function/1(distMP)
  MATLAB Function/1(HighTRFC) -> Switch/2
  Constant57/1 -> Switch/1
  Switch/1 -> HDV_Mu/1

== system HDVPSG_DelayComp_NewRef_RealDrop_case1/Subsystem7/Enabled Subsystem1 ==
  Front_to_end : Inport
  Enable : EnablePort
  Front_to_end_PDR : Outport
  wires:
  Front_to_end/1 -> Front_to_end_PDR/1

== system HDVPSG_DelayComp_NewRef_RealDrop_case1/Subsystem7/Enabled Subsystem2 ==
  v_Front : Inport
  Enable : EnablePort
  v_Front_PDR : Outport
  wires:
  v_Front/1 -> v_Front_PDR/1

== system HDVPSG_DelayComp_NewRef_RealDrop_case1/Subsystem7/Enabled Subsystem3 ==
  a_Front : Inport
  Enable : EnablePort
  a_Front_PDR : Outport
  wires:
  a_Front/1 -> a_Front_PDR/1

== system HDVPSG_DelayComp_NewRef_RealDrop_case1/HDV2_control_withPDR_compen/Subsystem/Enabled and Triggered Subsystem1 ==
  Enable : EnablePort  StatesWhenEnabling=reset
  Add : Sum
  Constant : Constant  SampleTime=T_ADE
  Memory : Memory
  Lost_stop : Outport
  wires:
  Constant/1 -> Add/1
  Memory/1 -> Add/2
  Add/1 -> Lost_stop/1, Memory/1

== system HDVPSG_DelayComp_NewRef_RealDrop_case1/PSG1_control_withPDR_compen/Subsystem/Enabled and Triggered Subsystem1 ==
  Enable : EnablePort  StatesWhenEnabling=reset
  Add : Sum
  Constant : Constant  SampleTime=T_ADE
  Memory : Memory
  Lost_stop : Outport
  wires:
  Add/1 -> Memory/1, Lost_stop/1
  Memory/1 -> Add/2
  Constant/1 -> Add/1

== system HDVPSG_DelayComp_NewRef_RealDrop_case1/PSG2_control_withPDR_compen/Subsystem/Enabled and Triggered Subsystem1 ==
  Enable : EnablePort  StatesWhenEnabling=reset
  Add : Sum
  Constant : Constant  SampleTime=T_ADE
  Memory : Memory
  Lost_stop : Outport
  wires:
  Constant/1 -> Add/1
  Memory/1 -> Add/2
  Add/1 -> Lost_stop/1, Memory/1

== system HDVPSG_DelayComp_NewRef_RealDrop_case1/PSG3_control_withPDR_compen/Subsystem/Enabled and Triggered Subsystem1 ==
  Enable : EnablePort  StatesWhenEnabling=reset
  Add : Sum
  Constant : Constant  SampleTime=T_ADE
  Memory : Memory
  Lost_stop : Outport
  wires:
  Add/1 -> Memory/1, Lost_stop/1
  Memory/1 -> Add/2
  Constant/1 -> Add/1

== system HDVPSG_DelayComp_NewRef_RealDrop_case1/Subsystem1/PSG_first/Body Fixed Vehicle Dynamics ==
  Tdf : Inport
  Brake : Inport  Port=2
  deltaFR : Inport  Port=3
  deltaFL : Inport  Port=4
  slope : Inport  Port=5
  TRFC : Inport  Port=6
  V_ini : Inport  Port=7
  yaw_ini : Inport  Port=8
  vy_ini : Inport  Port=9
  8dof_vehicle : Subsystem
  Brakes : Subsystem
  Bus Creator{,2..4} (4 alike) : BusCreator  Inputs=4
  Bus Creator1 : BusCreator  Inputs=8
  Bus Creator5 : BusCreator  Inputs=3
  Bus Selector : BusSelector  OutputSignals=signal1,signal2,signal3,signal4
  Constant : Constant  Value=0
  Constant1 : Constant  Value=0
  Driving Resistance Subsystem : Subsystem
  Fz : Subsystem
  Magic Formula Tire Model1 : Subsystem
  "Tire Longitudinal Center Speed " : Subsystem
  Tire Sideslip Angle : Subsystem
  Unit Delay : UnitDelay  SampleTime=UT.Ts_Veh  HasFrameUpgradeWarning=on
  Unit Delay1 : UnitDelay  SampleTime=UT.Ts_Veh  HasFrameUpgradeWarning=on
  deltaFL1 : InportShadow  Port=4
  deltaFL2 : InportShadow  Port=4
  deltaFR1 : InportShadow  Port=3
  deltaFR2 : InportShadow  Port=3
  lamda slip ratio : Subsystem
  omegafl : Outport  VectorParamsAs1DForOutWhenUnconnected=off
  omegafr : Outport  Port=2  VectorParamsAs1DForOutWhenUnconnected=off
  omegarl : Outport  Port=3  VectorParamsAs1DForOutWhenUnconnected=off
  omegarr : Outport  Port=4  VectorParamsAs1DForOutWhenUnconnected=off
  ax : Outport  Port=5  VectorParamsAs1DForOutWhenUnconnected=off
  Vx : Outport  Port=6  VectorParamsAs1DForOutWhenUnconnected=off
  "Yaw Rate " : Outport  Port=7  VectorParamsAs1DForOutWhenUnconnected=off
  Yaw Angle : Outport  Port=8  VectorParamsAs1DForOutWhenUnconnected=off
  ay : Outport  Port=9  VectorParamsAs1DForOutWhenUnconnected=off
  Vy : Outport  Port=10  VectorParamsAs1DForOutWhenUnconnected=off
  Beta : Outport  Port=11  VectorParamsAs1DForOutWhenUnconnected=off
  Sideslip Angle Alpha : Outport  Port=12  VectorParamsAs1DForOutWhenUnconnected=off
  wires:
  Brakes/4(Tbrr) -> 8dof_vehicle/5(Tbrr)
  Brakes/3(Tbrl) -> 8dof_vehicle/4(Tbrl)
  Brakes/2(Tbfr) -> 8dof_vehicle/3(Tbfr)
  Brakes/1(Tbfl) -> 8dof_vehicle/2(Tbfl)
  Brake/1 -> Brakes/2(brake postion)
  8dof_vehicle/14("Roll ") -> Fz/7(roll angle)
  8dof_vehicle/12(Pitch) -> Fz/4(pitch angle)
  8dof_vehicle/13(Pitch_rate) -> Fz/8(pitch rate)
  Bus Creator3/1 -> Bus Creator5/2
  deltaFR2/1 -> 8dof_vehicle/11(deltaRL)
  deltaFR1/1 -> Tire Sideslip Angle/5(deltaFR1)
  deltaFR/1 -> lamda slip ratio/10(deltaFR)
  lamda slip ratio/4(lamdarr) -> Bus Creator2/4
  lamda slip ratio/3(lamdarl) -> Bus Creator2/3
  lamda slip ratio/2(lamdafr) -> Bus Creator2/2
  lamda slip ratio/1(lamdafl) -> Bus Creator2/1
  Unit Delay/1 -> Fz/2(ax)
  Unit Delay1/1 -> Fz/5(ay)
  Magic Formula Tire Model1/4(Fy_FR) -> Bus Creator1/4
  Magic Formula Tire Model1/3(Fx_FR) -> Bus Creator1/3
  Magic Formula Tire Model1/6(Fy_RL) -> Bus Creator1/6
  Magic Formula Tire Model1/8(Fy_RR) -> Bus Creator1/8
  Magic Formula Tire Model1/7(Fx_RR) -> Bus Creator1/7
  Magic Formula Tire Model1/5(Fx_RL) -> Bus Creator1/5
  deltaFL2/1 -> 8dof_vehicle/10(deltaFL)  "deltaw"
  8dof_vehicle/5(ax) -> Unit Delay/1, ax/1
  Constant/1 -> Fz/3(slope)
  Driving Resistance Subsystem/1(Fax) -> 8dof_vehicle/7(Fax), Fz/1(Fa)
  Constant1/1 -> Fz/6(bank angle)
  slope/1 -> 8dof_vehicle/9(slope)
  8dof_vehicle/7(Yaw Rate) -> "Tire Longitudinal Center Speed "/3(YawRate), Tire Sideslip Angle/2(Yaw Rate), "Yaw Rate "/1
  8dof_vehicle/6(Vx) -> "Tire Longitudinal Center Speed "/1(Vx), Tire Sideslip Angle/3(Vx), Driving Resistance Subsystem/1(Vx), Vx/1
  8dof_vehicle/11("Veh Sideslip, Beta") -> Tire Sideslip Angle/6(Beta), Beta/1, "Tire Longitudinal Center Speed "/4(VehSideSlip Beta)
  8dof_vehicle/9(ay) -> Unit Delay1/1, ay/1
  deltaFL1/1 -> Tire Sideslip Angle/4(deltaFL)  "deltaw"
  deltaFL/1 -> lamda slip ratio/9(deltaFL)  "deltaw"
  Driving Resistance Subsystem/2(Fr) -> 8dof_vehicle/8(Fr)
  Bus Selector/4 -> lamda slip ratio/8(Vwrr)  "<signal4>"
  Bus Selector/3 -> lamda slip ratio/7(Vwrl)  "<signal3>"
  Bus Selector/2 -> lamda slip ratio/6(Vwfr)  "<signal2>"
  Bus Selector/1 -> lamda slip ratio/5(Vwfl)  "<signal1>"
  "Tire Longitudinal Center Speed "/3(Vwrl) -> Bus Creator/3
  "Tire Longitudinal Center Speed "/1(Vwfl) -> Bus Creator/1
  "Tire Longitudinal Center Speed "/2(Vwfr) -> Bus Creator/2
  "Tire Longitudinal Center Speed "/4(Vwrr) -> Bus Creator/4
  Tire Sideslip Angle/2(alpha_fr: rad) -> Bus Creator4/2
  Tire Sideslip Angle/1(alpha_fl: rad) -> Sideslip Angle Alpha/1, Bus Creator4/1
  Tire Sideslip Angle/3(alpha_rl: rad) -> Bus Creator4/3
  Tire Sideslip Angle/4(alpha_rr: rad) -> Bus Creator4/4
  Bus Creator5/1 -> Magic Formula Tire Model1/1(VehState)
  Bus Creator4/1 -> Bus Creator5/3  "alpha"
  Bus Creator2/1 -> Brakes/1(lambda), Bus Creator5/1  "lamda"
  Fz/1(Fzfl) -> Bus Creator3/1
  Fz/2(Fzfr) -> Bus Creator3/2
  Fz/3(Fzrl) -> Bus Creator3/3
  Fz/4(Fzrr) -> Bus Creator3/4
  Magic Formula Tire Model1/1(Fx_FL) -> Bus Creator1/1
  Magic Formula Tire Model1/2(Fy_FL) -> Bus Creator1/2
  8dof_vehicle/10(Vy) -> "Tire Longitudinal Center Speed "/2(Vy), Tire Sideslip Angle/1(Vy), Vy/1
  Bus Creator1/1 -> 8dof_vehicle/6(In7)
  8dof_vehicle/8(Yaw angle) -> Yaw Angle/1
  8dof_vehicle/4(omegarr) -> lamda slip ratio/4(omegarr), omegarr/1
  8dof_vehicle/3(omegarl) -> lamda slip ratio/3(omegarl), omegarl/1
  8dof_vehicle/2(omegafr) -> lamda slip ratio/2(omegafr), omegafr/1
  8dof_vehicle/1(omegafl) -> lamda slip ratio/1(omegafl), omegafl/1
  Tdf/1 -> 8dof_vehicle/1(Tdf)
  Bus Creator/1 -> Bus Selector/1
  TRFC/1 -> Magic Formula Tire Model1/2(TRFC)
  V_ini/1 -> 8dof_vehicle/12(V_ini)
  yaw_ini/1 -> 8dof_vehicle/13(yaw_ini)
  vy_ini/1 -> 8dof_vehicle/14(vy_ini)
  8dof_vehicle/15(Roll Rate) -> Fz/9(roll rate)

== system HDVPSG_DelayComp_NewRef_RealDrop_case1/Subsystem1/PSG_first/Cruise Speed Control ==
  Vx : Inport
  Vxr : Inport  Port=2
  PID_P : Inport  Port=3
  PID_I : Inport  Port=4
  PID_D : Inport  Port=5
  Constant : Constant  Value=100
  Gain : Gain  Gain=2
  PID Controller : simulink/Continuous/PID Controller  Controller=PID  Form=Parallel  TimeDomain=Discrete-time  SampleTime=UT.Ts_Veh  IntegratorMethod=Forward Euler  FilterMethod=Forward Euler  ControllerParametersSource=external  P=UT.PID_P_PSG  I=UT.PID_I_PSG  D=UT.PID_D_PSG  UseFilter=on  N=100  TunerSelectOption=Transfer Function Based (PID Tuner App)  InitialConditionSource=internal  InitialConditionForIntegrator=0  InitialConditionForFilter=0  DifferentiatorICPrevScaledInput=0  ExternalReset=none  TrackingMode=off  Kt=1  LimitOutput=off  UpperSaturationLimit=inf  LowerSaturationLimit=-inf  LinearizeAsGain=on  AntiWindupMode=none  Kb=1  POutMin=[]  POutMax=[]  IOutMin=[]  IOutMax=[]  DOutMin=[]  DOutMax=[]  NOutMin=[]  NOutMax=[]  SumOutMin=[]  SumOutMax=[]  SaturationOutMin=[]  SaturationOutMax=[]  PParamMin=[]  PParamMax=[]  IParamMin=[]  IParamMax=[]  DParamMin=[]  DParamMax=[]  NParamMin=[]  NParamMax=[]  KbParamMin=[]  KbParamMax=[]  KtParamMin=[]  KtParamMax=[]  KbOutMin=[]  KbOutMax=[]  KtOutMin=[]  KtOutMax=[]  IntegratorOutMin=[]  IntegratorOutMax=[]  FilterOutMin=[]  FilterOutMax=[]  SumI1OutMin=[]  SumI1OutMax=[]  SumI2OutMin=[]  SumI2OutMax=[]  SumI3OutMin=[]  SumI3OutMax=[]  SumI4OutMin=[]  SumI4OutMax=[]  SumDOutMin=[]  SumDOutMax=[]  DifferentiatorOutMin=[]  DifferentiatorOutMax=[]  FilterDiffOutCoefMin=[]  FilterDiffOutCoefMax=[]  ReciprocalOutMin=[]  ReciprocalOutMax=[]  SumDenOutMin=[]  SumDenOutMax=[]  SumNumOutMin=[]  SumNumOutMax=[]  DivideOutMin=[]  DivideOutMax=[]  IntegratorContinuousStateAttributes=''  IntegratorStateMustResolveToSignalObject=off  IntegratorRTWStateStorageClass=Auto  FilterContinuousStateAttributes=''  FilterStateMustResolveToSignalObject=off  FilterRTWStateStorageClass=Auto  ParallelPVariant=ExternalParameters  IdealPVariant=Disabled  IVariant=ExternalParameters  DVariant=ExternalParameters  IntegratorVariant=Discrete  SatVariant=Disabled  AWVariant=Passthrough  PCopyVariant=Disabled  TRVariant=Disabled  FdbkBlocksVariant=Forward  IdealPFdbkVariant=Disabled  SatFdbkVariant=Disabled  DerivativeFilterVariant=ForwardEulerFilter  NVariant=ExternalParameters  NCopyVariant=Disabled  FilterICVariant=InternalICsFilter  IntegratorICVariant=InternalICs  ExternalResetVariant=Disabled  TRSumVariant=Passthrough  SumFdbkVariant=Disabled  SumVariant=Sum_PID
  Subtract : Sum  Inputs=-+
  Throttle : Outport  VectorParamsAs1DForOutWhenUnconnected=off
  wires:
  Vx/1 -> Subtract/1
  Vxr/1 -> Subtract/2
  Gain/1 -> Throttle/1
  Subtract/1 -> PID Controller/1
  PID Controller/1 -> Gain/1
  Constant/1 -> PID Controller/5
  PID_P/1 -> PID Controller/2
  PID_I/1 -> PID Controller/3
  PID_D/1 -> PID Controller/4
